simulink model "Example"

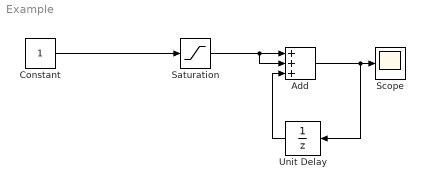
== system Example ==
  Add : Sum  Inputs=+++
  Constant : Constant
  Saturation : Saturate
  Scope : Scope
  Unit Delay : UnitDelay  SampleTime=-1  HasFrameUpgradeWarning=on
  wires:
  Constant/1 -> Saturation/1
  Saturation/1 -> Add/2, Add/1
  Add/1 -> Unit Delay/1, Scope/1
  Unit Delay/1 -> Add/3
